simulink model "ControlLogic_pho"  (R2019a)
settings: Solver=FixedStepAuto  StartTime=0.0  StopTime=86400  FixedStep=3600  RelTol=1e-3
libraries: simulink x7
settings Model: Creator=Administrator  LastModifiedBy=Administrator

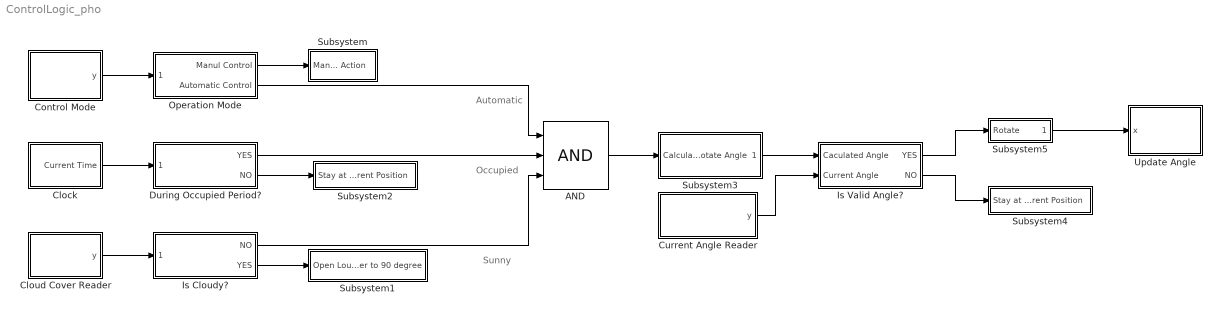
== system ControlLogic_pho ==
  note: Automatic
  note: Occupied
  note: Sunny
  AND : Logic  Inputs=3  IconShape=distinctive  AllPortsSameDT=off  OutDataTypeStr=boolean
  Clock : Subsystem
  "Cloud Cover Reader " : MATLAB Function  TreatAsAtomicUnit=on
  Control Mode : MATLAB Function  TreatAsAtomicUnit=on
  "Current Angle Reader " : MATLAB Function  TreatAsAtomicUnit=on
  During Occupied Period? : Subsystem
  Is Cloudy? : Subsystem
  Is Valid Angle? : Subsystem
  Operation Mode : Subsystem
  Subsystem : Subsystem
  Subsystem1 : Subsystem
  Subsystem2 : Subsystem
  Subsystem3 : Subsystem
  Subsystem4 : Subsystem
  Subsystem5 : Subsystem
  Update Angle : MATLAB Function  TreatAsAtomicUnit=on
  wires:
  "Cloud Cover Reader "/1(y) -> Is Cloudy?/1(" ")
  Clock/1(Current Time) -> During Occupied Period?/1(" ")
  AND/1 -> Subsystem3/1(Calculate Rotate Angle)
  "Current Angle Reader "/1(y) -> Is Valid Angle?/2(Current Angle)
  Is Cloudy?/2("YES ") -> Subsystem1/1(" Open Louver to 90 degree")
  Operation Mode/1("Manul Control ") -> Subsystem/1(Manual Action)
  Control Mode/1(y) -> Operation Mode/1(" ")
  During Occupied Period?/2("NO ") -> Subsystem2/1(Stay at Current Position)
  Operation Mode/2(Automatic Control) -> AND/1
  During Occupied Period?/1(YES) -> AND/2
  Is Cloudy?/1(NO) -> AND/3
  Subsystem3/1(" ") -> Is Valid Angle?/1(Caculated Angle)
  Subsystem5/1("  ") -> Update Angle/1(x)
  Is Valid Angle?/2("NO ") -> Subsystem4/1(Stay at Current Position)
  Is Valid Angle?/1(YES) -> Subsystem5/1(Rotate)

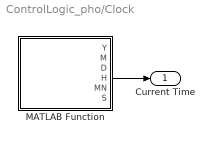
== system ControlLogic_pho/Clock ==
  MATLAB Function : MATLAB Function  TreatAsAtomicUnit=on
  Current Time : Outport
  wires:
  MATLAB Function/4(H) -> Current Time/1

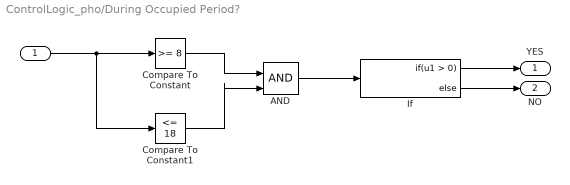
== system ControlLogic_pho/During Occupied Period? ==
  " " : Inport
  AND : Logic  IconShape=distinctive  AllPortsSameDT=off  OutDataTypeStr=boolean
  Compare To Constant : simulink/Logic and Bit Operations/Compare To Constant  relop=>=  const=8  OutDataTypeStr=boolean
  Compare To Constant1 : simulink/Logic and Bit Operations/Compare To Constant  relop=<=  const=18  OutDataTypeStr=boolean
  If : If
  YES : Outport
  "NO " : Outport  Port=2
  wires:
  Compare To Constant1/1 -> AND/2
  Compare To Constant/1 -> AND/1
  " "/1 -> Compare To Constant1/1, Compare To Constant/1
  AND/1 -> If/1
  If/1 -> YES/1
  If/2 -> "NO "/1

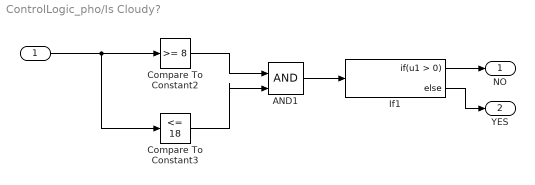
== system ControlLogic_pho/Is Cloudy? ==
  " " : Inport
  AND1 : Logic  IconShape=distinctive  AllPortsSameDT=off  OutDataTypeStr=boolean
  Compare To Constant2 : simulink/Logic and Bit Operations/Compare To Constant  relop=>=  const=8  OutDataTypeStr=boolean
  Compare To Constant3 : simulink/Logic and Bit Operations/Compare To Constant  relop=<=  const=18  OutDataTypeStr=boolean
  If1 : If
  NO : Outport
  "YES " : Outport  Port=2
  wires:
  " "/1 -> Compare To Constant3/1, Compare To Constant2/1
  Compare To Constant3/1 -> AND1/2
  Compare To Constant2/1 -> AND1/1
  AND1/1 -> If1/1
  If1/1 -> NO/1
  If1/2 -> "YES "/1

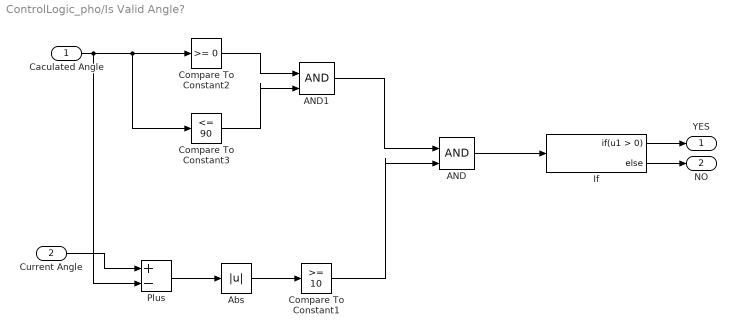
== system ControlLogic_pho/Is Valid Angle? ==
  Caculated Angle : Inport
  Current Angle : Inport  Port=2
  AND : Logic  IconShape=distinctive  AllPortsSameDT=off  OutDataTypeStr=boolean
  AND1 : Logic  IconShape=distinctive  AllPortsSameDT=off  OutDataTypeStr=boolean
  Abs : Abs
  Compare To Constant1 : simulink/Logic and Bit Operations/Compare To Constant  relop=>=  const=10  OutDataTypeStr=boolean
  Compare To Constant2 : simulink/Logic and Bit Operations/Compare To Constant  relop=>=  const=0  OutDataTypeStr=boolean
  Compare To Constant3 : simulink/Logic and Bit Operations/Compare To Constant  relop=<=  const=90  OutDataTypeStr=boolean
  If : If
  Plus : Sum  Inputs=+-
  YES : Outport
  "NO " : Outport  Port=2
  wires:
  AND1/1 -> AND/1
  Caculated Angle/1 -> Plus/2, Compare To Constant3/1, Compare To Constant2/1
  Compare To Constant3/1 -> AND1/2
  Compare To Constant2/1 -> AND1/1
  Current Angle/1 -> Plus/1
  Plus/1 -> Abs/1
  Abs/1 -> Compare To Constant1/1
  Compare To Constant1/1 -> AND/2
  AND/1 -> If/1
  If/1 -> YES/1
  If/2 -> "NO "/1

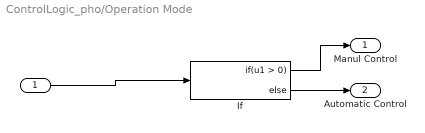
== system ControlLogic_pho/Operation Mode ==
  " " : Inport
  If : If
  "Manul Control " : Outport
  Automatic Control : Outport  Port=2
  wires:
  If/1 -> "Manul Control "/1
  If/2 -> Automatic Control/1
  " "/1 -> If/1

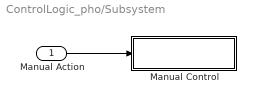
== system ControlLogic_pho/Subsystem ==
  Manual Action : Inport
  Manual Control : Subsystem  TreatAsAtomicUnit=on
  wires:
  Manual Action/1 -> Manual Control/Action

== system ControlLogic_pho/Subsystem1 ==
  " Open Louver to 90 degree" : Inport
  Action : Subsystem  TreatAsAtomicUnit=on
  wires:
  " Open Louver to 90 degree"/1 -> Action/Action

== system ControlLogic_pho/Subsystem2 ==
  Stay at Current Position : Inport

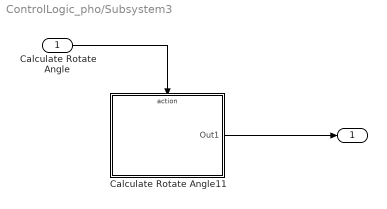
== system ControlLogic_pho/Subsystem3 ==
  Calculate Rotate Angle : Inport
  Calculate Rotate Angle11 : Subsystem  TreatAsAtomicUnit=on
  " " : Outport
  wires:
  Calculate Rotate Angle/1 -> Calculate Rotate Angle11/Action
  Calculate Rotate Angle11/1(Out1) -> " "/1

== system ControlLogic_pho/Subsystem4 ==
  Stay at Current Position : Inport

== system ControlLogic_pho/Subsystem5 ==
  Rotate : Inport
  "  " : Outport

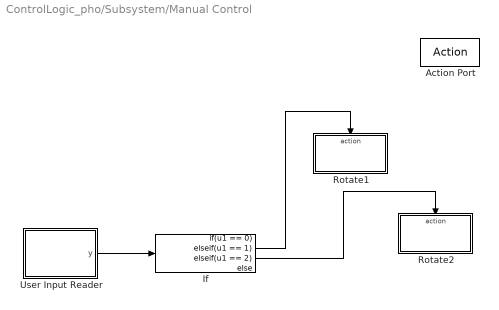
== system ControlLogic_pho/Subsystem/Manual Control ==
  Action Port : ActionPort  ActionPortLabel=if(u1 > 0)
  If : If  IfExpression=u1 == 0  ElseIfExpressions=u1 == 1, u1 == 2
  Rotate1 : Subsystem  TreatAsAtomicUnit=on
  Rotate2 : Subsystem  TreatAsAtomicUnit=on
  User Input Reader : MATLAB Function  TreatAsAtomicUnit=on
  wires:
  User Input Reader/1(y) -> If/1
  If/2 -> Rotate1/Action
  If/3 -> Rotate2/Action

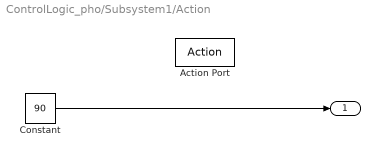
== system ControlLogic_pho/Subsystem1/Action ==
  Action Port : ActionPort  ActionPortLabel=else
  Constant : Constant  Value=90
  " " : Outport
  wires:
  Constant/1 -> " "/1

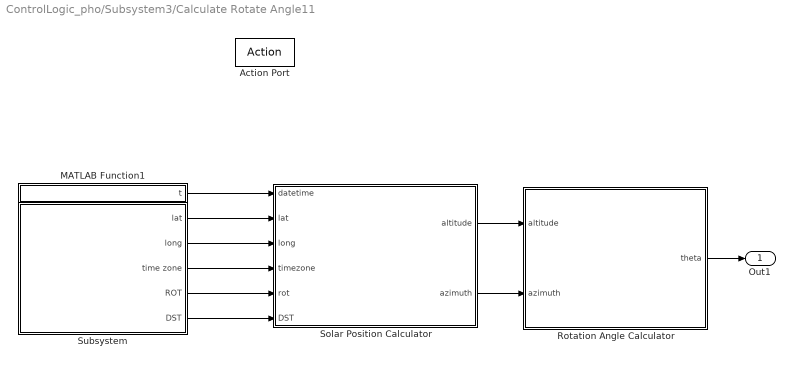
== system ControlLogic_pho/Subsystem3/Calculate Rotate Angle11 ==
  Action Port : ActionPort
  MATLAB Function1 : MATLAB Function  TreatAsAtomicUnit=on
  Rotation Angle Calculator : MATLAB Function  TreatAsAtomicUnit=on
  Solar Position Calculator : MATLAB Function  TreatAsAtomicUnit=on
  Subsystem : Subsystem
  Out1 : Outport
  wires:
  Solar Position Calculator/1(altitude) -> Rotation Angle Calculator/1(altitude)
  Subsystem/5(DST) -> Solar Position Calculator/6(DST)
  Subsystem/4(ROT) -> Solar Position Calculator/5(rot)
  Subsystem/3(time zone) -> Solar Position Calculator/4(timezone)
  Subsystem/2(long) -> Solar Position Calculator/3(long)
  Subsystem/1(lat) -> Solar Position Calculator/2(lat)
  MATLAB Function1/1(t) -> Solar Position Calculator/1(datetime)
  Solar Position Calculator/2(azimuth) -> Rotation Angle Calculator/2(azimuth)
  Rotation Angle Calculator/1(theta) -> Out1/1

== system ControlLogic_pho/Subsystem/Manual Control/Rotate1 ==
  Action Port : ActionPort  ActionPortLabel=elseif(u1 == 1)
  MATLAB Function : MATLAB Function  TreatAsAtomicUnit=on

== system ControlLogic_pho/Subsystem/Manual Control/Rotate2 ==
  Action Port : ActionPort  ActionPortLabel=elseif( u1 == 2)
  MATLAB Function : MATLAB Function  TreatAsAtomicUnit=on

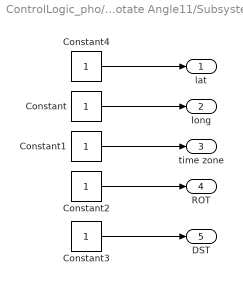
== system ControlLogic_pho/Subsystem3/Calculate Rotate Angle11/Subsystem ==
  Constant{,1..4} (5 alike) : Constant
  lat : Outport
  long : Outport  Port=2
  time zone : Outport  Port=3
  ROT : Outport  Port=4
  DST : Outport  Port=5
  wires:
  Constant4/1 -> lat/1
  Constant/1 -> long/1
  Constant1/1 -> time zone/1
  Constant2/1 -> ROT/1
  Constant3/1 -> DST/1

== matlab function ControlLogic_pho/Subsystem3/Calculate Rotate Angle11/MATLAB Function1 ==
  data: t output
function t = fcn()
   coder.extrinsic('now');
   coder.extrinsic('datevec');
   Y = 0;
   M = 0;
   D = 0;
   H = 0;
   MN = 0;
   S = 0;
   [Y, M, D, H, MN, S] = datevec(now);
   t = [Y, M, D, H, MN, S];
end

== matlab function ControlLogic_pho/Subsystem3/Calculate Rotate Angle11/Solar Position Calculator ==
  data: datetime input; altitude output; lat input; long input; timezone input; rot input; DST input; azimuth output
function [altitude, azimuth] = position(datetime,lat,long,timezone,rot,DST)
altitude = 42;
azimuth = 42;

== matlab function ControlLogic_pho/Cloud Cover Reader  ==
  data: y output
function y = cloud_cover()
coder.extrinsic("xlsread");
y = 0;
%coder.extrinsic('y');

y = xlsread("weather.csv", 'B27:B27');

== matlab function ControlLogic_pho/Current Angle Reader  ==
  data: y output
function y = read()
coder.extrinsic("csvread");
y = 0;
%coder.extrinsic('y');

y = csvread("test.csv");

== matlab function ControlLogic_pho/Subsystem/Manual Control/Rotate1/MATLAB Function ==
  data: y output
%function y = fcn(u)

%y = u;
function y = fcn()
system('bacwp.exe 701103 4 6 85 8 -1 9 1');
pause(4);
system('bacwp.exe 701103 4 6 85 8 -1 9 0');
y = 1;
end

== matlab function ControlLogic_pho/Update Angle ==
  data: x input
function update(x)
coder.extrinsic("csvread");

== matlab function ControlLogic_pho/Subsystem3/Calculate Rotate Angle11/Rotation Angle Calculator ==
  data: altitude input; theta output; azimuth input
function theta = calculator(altitude,azimuth)

theta = 42;

== matlab function ControlLogic_pho/Control Mode ==
  data: y output
function y = mode()
coder.extrinsic("xlsread");
y = 0;
%coder.extrinsic('y');

y = xlsread("node.csv", 'A1:A1');

== matlab function ControlLogic_pho/Clock/MATLAB Function ==
  data: Y output; M output; D output; H output; MN output; S output
function [Y, M, D, H, MN, S] = fcn()
   coder.extrinsic('now');
   coder.extrinsic('datevec');
   Y = 0;
   M = 0;
   D = 0;
   H = 0;
   MN = 0;
   S = 0;
   [Y, M, D, H, MN, S] = datevec(now);
end

== matlab function ControlLogic_pho/Subsystem/Manual Control/Rotate2/MATLAB Function ==
  data: y output
%function y = fcn(u)

%y = u;
function y = fcn()
system('bacwp.exe 701103 4 7 85 8 -1 9 1');
pause(4);
system('bacwp.exe 701103 4 7 85 8 -1 9 0');
y = 1;
end

== matlab function ControlLogic_pho/Subsystem/Manual Control/User Input Reader ==
  data: y output
 function y = fcn()
coder.extrinsic("csvread");
y = 0;
%coder.extrinsic('y');

y = xlsread("test_1.csv","A1:A1");
